simulink model "sim_battery_testrack_"  (R2023a)
settings: configuration reference "SharedConfig" (kept outside this file)
undefined symbols (not defined in the file or in its folder): battery_builder_rtmsupport, gcbh
libraries: nesl_utility x14, GD_Batterymodel_6_lib x8, fl_lib x7, BatteryCurrentManagement x1, batt_lib x1, BatteryBalancing x1, simulink x1, SimscapeFluids_lib x1
(part 1 of 2)
settings Model: Creator=DM  LastModifiedBy=ga84jar
settings ConfigSetRef: SourceName=SharedConfig  SourceLocation=Base Workspace

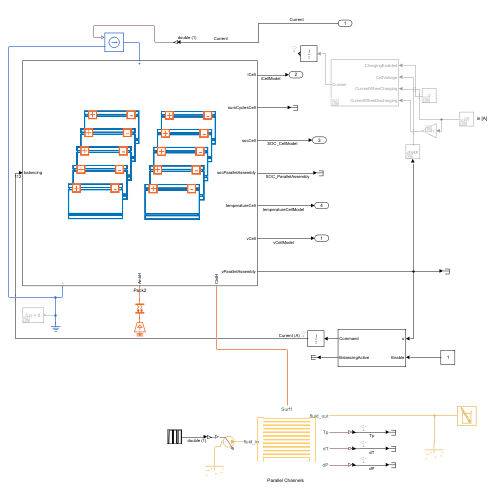
[thumbnail: Simulink's stored preview of the top-level diagram]
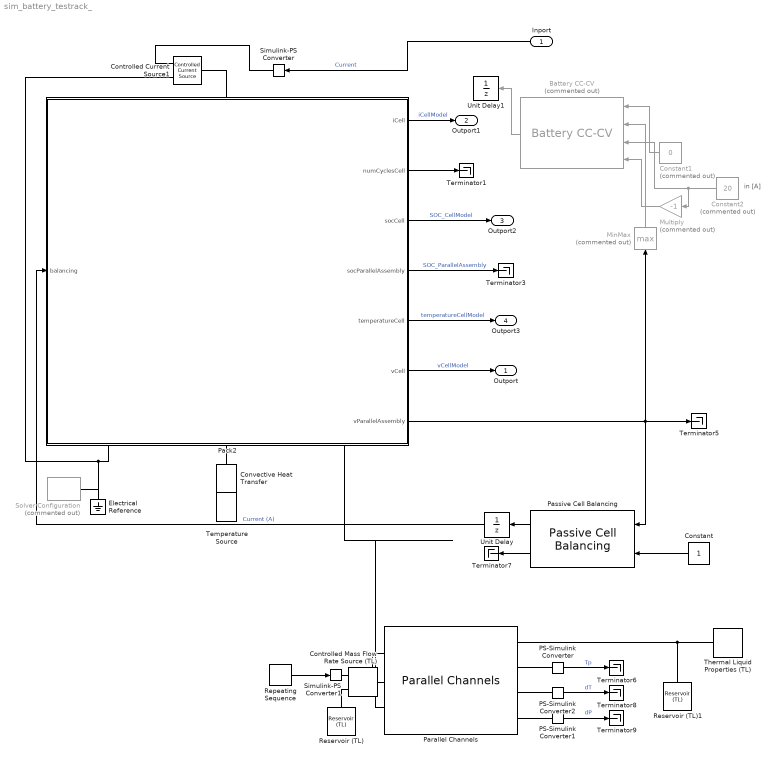
== system sim_battery_testrack_ ==
  note: in [A]
  Inport : Inport
  Battery CC-CV : BatteryCurrentManagement/Battery CC-CV  Commented=on  MaxCellVoltage=4.5  Kp=100  Ki=10  Kaw=1  Kt=1  Ts=-1
      settings: LibrarySourceBlock=batt_sl_lib/Current Management/Battery CC-CV
  Constant : Constant
  Constant1 : Constant  Commented=on  Value=0
  Constant2 : Constant  Commented=on  Value=20
  Controlled Current Source1 : fl_lib/Electrical/Electrical Sources/Controlled Current Source
  Controlled Mass Flow Rate Source (TL) : fl_lib/Thermal Liquid/Sources/Controlled Mass Flow Rate Source (TL)  power_spec=foundation.enum.power_spec.isentropic  area=0.01 m^2
      settings: InternalSimscapePortConfiguration="{\"Bottom\":[],\"Left\":[{\"id\":\"A\",\"label\":\"A\",\"type\":\"foundation.thermal_liquid.thermal_liquid\"},{\"id\":\"M\",\"label\":\"M\",\"type\":\"input\"}],\"Right\":[{\"id\":\"B\",\"label\":\"B\",\"type\":\"foundation.thermal_liquid.thermal_liquid\"}],\"Top\":[]}"
  Convective Heat Transfer : fl_lib/Thermal/Thermal Elements/Convective Heat Transfer  thermal_type=foundation.enum.constant_variable.constant  area=1e-4 m^2  heat_tr_coeff=20 W/(K*m^2)  min_heat_tr_coeff=1e-3 W/(K*m^2)  T_specify=off  T_priority=None  T=0 K  T_nominal_specify=off  T_nominal_unit=K  T_nominal_value=1  Q_specify=off  Q_priority=None  Q=0 W  Q_nominal_specify=off  Q_nominal_unit=W  Q_nominal_value=1
  Electrical Reference : fl_lib/Electrical/Electrical Elements/Electrical Reference
  MinMax : MinMax  Commented=on  Function=max
  Multiply : Gain  Commented=on  Gain=-1
  PS-Simulink Converter : nesl_utility/PS-Simulink Converter  PhysicalDomain=network_engine_domain  SubClassName=ps_output  LeftPortType=input  RightPortType=output  PseudoPeriodic=off  Frequencies=[]  VectorFormat=inherit  Unit=inherit  AffineConversion=off
  PS-Simulink Converter1 : nesl_utility/PS-Simulink Converter  PhysicalDomain=network_engine_domain  SubClassName=ps_output  LeftPortType=input  RightPortType=output  PseudoPeriodic=off  Frequencies=[]  VectorFormat=inherit  Unit=inherit  AffineConversion=off
  PS-Simulink Converter2 : nesl_utility/PS-Simulink Converter  PhysicalDomain=network_engine_domain  SubClassName=ps_output  LeftPortType=input  RightPortType=output  PseudoPeriodic=off  Frequencies=[]  VectorFormat=inherit  Unit=inherit  AffineConversion=off
  Pack2 : Subsystem  LoadFcn=battery_builder_rtmsupport('loadfcn',gcbh);
      settings: CopyFcn=battery_builder_rtmsupport('copyfcn',gcbh);  PreCopyFcn=battery_builder_rtmsupport('precopyfcn',gcbh);  PreDeleteFcn=battery_builder_rtmsupport('predeletefcn',gcbh);  PortSchema="{\"entries\":[{\"content\":{\"sides\":[{\"content\":{\"connectorIds\":[\"LConn1\"]},\"type\":\"ConnectorPlacement.EquallySpacedRectSide\",\"uuid\":\"eaf430c6-d28e-4a62-8b49-4d37c8edca5f\"},{\"content\":{\"connectorIds\":[\"RConn1\",\"RConn2\",\"RConn3\"],\"side\":\"RIGHT\"},\"type\":\"ConnectorPlacement.EquallySpacedRectSide\",\"uuid\":\"a95fddc1-7334-484a-9b4b-2e1f2360c9bb\"},{\"content\":{\"connectorIds\":[\"In1\"],\"side\":\"TOP\"},\"type\":\"ConnectorPlacement.EquallySpacedRectSide\",\"uuid\":\"f8c05a41-d443-4265-a433-e5e7047f73b2\"},{\"content\":{\"connectorIds\":[\"Out1\",\"Out2\",\"Out3\",\"Out4\",\"Out5\",\"Out6\",\"Out7\"],\"side\":\"BOTTOM\"},\"type\":\"ConnectorPlacement.EquallySpacedRectSide\",\"uuid\":\"9eaec147-65ce-4588-accb-be47b4d057de\"}]},\"type\":\"ConnectorPlacement.EquallySpacedConnector\",\"uuid\":\"9deafdf2-66e7-49dd-9ff8-5fa03867202c\"}],\"packageUris\":[\"http://schema.mathworks.com/mf0/Connector/R2020b\"],\"version\":\"1.0\"}"
      mask Display: image('$imagefile')
  Parallel Channels : batt_lib/Thermal/Parallel Channels  plateConnectivity=simscape.battery.enum.thermal.coolingPlateConnectivity.singleSided  numBattThermalNodes1=1  dimensionThermalNodes1=ones(1, 2)  locationThermalNodes1=ones(1, 2)  numBattThermalNodes2=1  dimensionThermalNodes2=ones(1, 2)  locationThermalNodes2=ones(1, 2)  plateDimX=2  plateDimY=5  plateTh=2e-3 m  plateThCond=20 W/(K*m)  plateDen=2500 kg/m^3  plateCp=447 J/(K*kg)  plateTemp_ini=300 K  Re_lam=2000  Re_tur=4000  Nu_lam=3.66  length_add=1e-3 m  shape_factor=64  nChannels=4  selectChannelOrientation=simscape.battery.enum.thermal.coolingChannelsDirection.alongX  channelDia=0.005 m  distributorDia=0.005 m  roughnessPipe=1.5e-05 m
      settings: InternalSimscapePortConfiguration="{\"Bottom\":[],\"Left\":[{\"id\":\"fluid_in\",\"label\":\"fluid_in\",\"type\":\"foundation.thermal_liquid.thermal_liquid\"}],\"Right\":[{\"id\":\"fluid_out\",\"label\":\"fluid_out\",\"type\":\"foundation.thermal_liquid.thermal_liquid\"},{\"id\":\"plotPlateT\",\"label\":\"Tp\",\"type\":\"output\"},{\"id\":\"tempSensor\",\"label\":\"dT\",\"type\":\"output\"},{\"id\":\"presSensor\",\"label\":\"dP\",\"type\":\"output\"}],\"Top\":[{\"id\":\"Side1\",\"label\":\"Surf1\",\"type\":\"foundation.thermal.thermal\"}]}"
  Passive Cell Balancing : BatteryBalancing/Passive Cell Balancing  Threshold=0.2  Td_on=1  Td_off=1  Ts=-1  dataType=double
      settings: LibrarySourceBlock=batt_sl_lib/Cell Balancing/Passive Cell Balancing
  Repeating Sequence : simulink/Sources/Repeating Sequence  rep_seq_t=[0 500 550 2001]  rep_seq_y=[0.00 0.00 0.01 0.01]
  Reservoir (TL) : fl_lib/Thermal Liquid/Elements/Reservoir (TL)  pressure_spec=foundation.enum.pressure_spec.atmospheric  reservoir_pressure=0.101325 MPa  reservoir_temperature=293.15 K  area=0.01 m^2
  Reservoir (TL)1 : fl_lib/Thermal Liquid/Elements/Reservoir (TL)  pressure_spec=foundation.enum.pressure_spec.atmospheric  reservoir_pressure=0.101325 MPa  reservoir_temperature=293.15 K  area=0.01 m^2
  Simulink-PS Converter : nesl_utility/Simulink-PS Converter  PhysicalDomain=network_engine_domain  SubClassName=ps_input  LeftPortType=input  RightPortType=output  PseudoPeriodic=off  Frequencies=[]  NoiseDistribution=none  NoiseParameters=[]  Unit=1  AffineConversion=off  FilteringAndDerivatives=provide  SimscapeFilterOrder=1  InputFilterTimeConstant=0.001  UdotUserProvided=0
  Simulink-PS Converter1 : nesl_utility/Simulink-PS Converter  PhysicalDomain=network_engine_domain  SubClassName=ps_input  LeftPortType=input  RightPortType=output  PseudoPeriodic=off  Frequencies=[]  NoiseDistribution=none  NoiseParameters=[]  Unit=1  AffineConversion=off  FilteringAndDerivatives=provide  SimscapeFilterOrder=1  InputFilterTimeConstant=0.001  UdotUserProvided=0
  Solver Configuration : nesl_utility/Solver Configuration  Commented=on  PhysicalDomain=network_engine_domain  SubClassName=solver  LeftPortType=input  RightPortType=generic  Tones=[]  Harmonics=[]  SimulateNoise=off  Profile=off  UseLocalSampling=off  EnableSwitchedLinearOptims=on  FrequencyDomain=off  UseCCode=off  RelTol=0.001  AbsTol=0.001  MinStep=1e-09  ToWorkspace=off  RevertToSquareIcSolve=off  NumHomotopyIterations=100  PhasorMode=off  PhasorModeNumHarmonics=1  ConsistencySolver=NEWTON_XTOL_AFTER_FTOL  IndexReductionMethod=DerivativeReplacement  DoDC=off  ResidualTolerance=1e-09  ConsistencyTolSource=GLOBAL  ConsistencyAbsTol=0.001  ConsistencyRelTol=0.001  ConsistencyTolFactor=0.001  UseLocalSolver=on  LocalSolverChoice=NE_BACKWARD_EULER_ADVANCER  ResolveIndetEquations=on  FunctionEvalNumThread=1  LocalSolverSampleTime=1  DoFixedCost=on  MaxNonlinIter=3  MaxModeIter=2  ComputeImpulses=off  ImpulseIterations=2  LinearAlgebra=auto  LinearAlgebraNumThread=0  EquationFormulation=NE_TIME_EF  DelaysMemoryBudget=51200  AutomaticFiltering=on  FilteringTimeConstant=0.001  PartitionStorageMethod=AS_NEEDED  PartitionMemoryBudget=1024  PartitionMethod=ROBUST
  Temperature Source : fl_lib/Thermal/Thermal Sources/Temperature Source  temperature=273.15+25 K
  Terminator{1,3,5..9} (7 alike) : Terminator
  Thermal Liquid Properties (TL) : SimscapeFluids_lib/Thermal Liquid/Utilities/Thermal Liquid Properties (TL)  fluid_list=fluids.thermal_liquid.utilities.enum.thermal_liquid_fluid_list.water  concentration_param_EG=fluids.thermal_liquid.utilities.enum.thermal_liquid_concentration.volume_fraction  concentration_param_PG=fluids.thermal_liquid.utilities.enum.thermal_liquid_concentration.volume_fraction  c_mass_SW=3.5e-3  c_mass_EG=0.1  c_mass_PG=0.1  c_mass_GL=0.1  c_vol_EG=0.1  c_vol_PG=0.1  beta_const_EG=2.1791 GPa  beta_const_PG=2.1791 GPa  beta_const_GL=2.1791 GPa  p_min_EG=0.01 MPa  p_min_PG=0.01 MPa  p_min_GL=0.01 MPa  p_max_EG=50 MPa  p_max_PG=50 MPa  p_max_GL=50 MPa  p_atm=0.101325 MPa  properties_range_check=simscape.enum.assert.action.error
  Unit Delay : UnitDelay  SampleTime=-1  HasFrameUpgradeWarning=on
  Unit Delay1 : UnitDelay  SampleTime=-1  HasFrameUpgradeWarning=on
  Outport : Outport
  Outport1 : Outport  Port=2
  Outport2 : Outport  Port=3
  Outport3 : Outport  Port=4
  wires:
  Pack2/1(iCell) -> Outport1/1  "iCellModel"
  Pack2/2(numCyclesCell) -> Terminator1/1
  Pack2/3(socCell) -> Outport2/1  "SOC_CellModel"
  Pack2/4(socParallelAssembly) -> Terminator3/1  "SOC_ParallelAssembly"
  Pack2/5(temperatureCell) -> Outport3/1  "temperatureCellModel"
  Pack2/6(vCell) -> Outport/1  "vCellModel"
  Passive Cell Balancing/2 -> Terminator7/1
  Constant/1 -> Passive Cell Balancing/2
  Constant1/1 -> Battery CC-CV/1
  Constant2/1 -> Multiply/1, Battery CC-CV/3
  Multiply/1 -> Battery CC-CV/4
  MinMax/1 -> Battery CC-CV/2
  Passive Cell Balancing/1 -> Unit Delay/1
  Unit Delay/1 -> Pack2/1(balancing)  "Current (A)"
  PS-Simulink Converter/1 -> Terminator6/1  "Tp"
  PS-Simulink Converter2/1 -> Terminator8/1  "dT"
  PS-Simulink Converter1/1 -> Terminator9/1  "dP"
  Repeating Sequence/1 -> Simulink-PS Converter1/1
  Inport/1 -> Simulink-PS Converter/1  "Current"
  Pack2/7(vParallelAssembly) -> Terminator5/1, Passive Cell Balancing/1, MinMax/1
  Battery CC-CV/1 -> Unit Delay1/1
  connections:
  Pack2/LConn1 -- Controlled Current Source1/LConn1
  Controlled Current Source1/RConn2 -- Pack2/RConn1 -- Electrical Reference/LConn1 -- Solver Configuration/RConn1
  Simulink-PS Converter/RConn1 -- Controlled Current Source1/RConn1
  Pack2/RConn3 -- Parallel Channels/LConn2
  PS-Simulink Converter/LConn1 -- Parallel Channels/RConn2
  PS-Simulink Converter2/LConn1 -- Parallel Channels/RConn3
  Parallel Channels/RConn4 -- PS-Simulink Converter1/LConn1
  Controlled Mass Flow Rate Source (TL)/RConn1 -- Parallel Channels/LConn1
  Simulink-PS Converter1/RConn1 -- Controlled Mass Flow Rate Source (TL)/LConn2
  Reservoir (TL)/LConn1 -- Controlled Mass Flow Rate Source (TL)/LConn1
  Thermal Liquid Properties (TL)/RConn1 -- Parallel Channels/RConn1 -- Reservoir (TL)1/LConn1
  Pack2/RConn2 -- Convective Heat Transfer/LConn1
  Temperature Source/LConn1 -- Convective Heat Transfer/RConn1

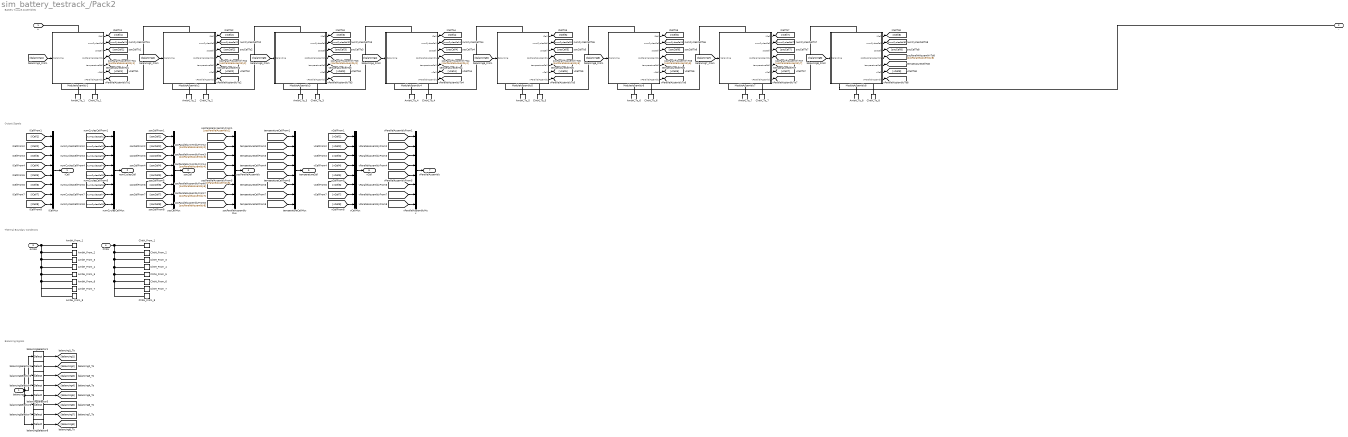
== system sim_battery_testrack_/Pack2 ==
  note: Battery Module Assemblies
  note: Output Signals
  note: Thermal Boundary Conditions
  note: Balancing Signals
  balancing : Inport  PortDimensions=112
  AmbH_From_1 : ConnectionLabel  Label=ambH_1
  AmbH_From_2 : ConnectionLabel  Label=ambH_2
  AmbH_From_3 : ConnectionLabel  Label=ambH_3
  AmbH_From_4 : ConnectionLabel  Label=ambH_4
  AmbH_From_5 : ConnectionLabel  Label=ambH_5
  AmbH_From_6 : ConnectionLabel  Label=ambH_6
  AmbH_From_7 : ConnectionLabel  Label=ambH_7
  AmbH_From_8 : ConnectionLabel  Label=ambH_8
  AmbH_To_1 : ConnectionLabel  Label=ambH_1
  AmbH_To_2 : ConnectionLabel  Label=ambH_2
  AmbH_To_3 : ConnectionLabel  Label=ambH_3
  AmbH_To_4 : ConnectionLabel  Label=ambH_4
  AmbH_To_5 : ConnectionLabel  Label=ambH_5
  AmbH_To_6 : ConnectionLabel  Label=ambH_6
  AmbH_To_7 : ConnectionLabel  Label=ambH_7
  AmbH_To_8 : ConnectionLabel  Label=ambH_8
  ClntH_From_1 : ConnectionLabel  Label=clntH_1
  ClntH_From_2 : ConnectionLabel  Label=clntH_2
  ClntH_From_3 : ConnectionLabel  Label=clntH_3
  ClntH_From_4 : ConnectionLabel  Label=clntH_4
  ClntH_From_5 : ConnectionLabel  Label=clntH_5
  ClntH_From_6 : ConnectionLabel  Label=clntH_6
  ClntH_From_7 : ConnectionLabel  Label=clntH_7
  ClntH_From_8 : ConnectionLabel  Label=clntH_8
  ClntH_To_1 : ConnectionLabel  Label=clntH_1
  ClntH_To_2 : ConnectionLabel  Label=clntH_2
  ClntH_To_3 : ConnectionLabel  Label=clntH_3
  ClntH_To_4 : ConnectionLabel  Label=clntH_4
  ClntH_To_5 : ConnectionLabel  Label=clntH_5
  ClntH_To_6 : ConnectionLabel  Label=clntH_6
  ClntH_To_7 : ConnectionLabel  Label=clntH_7
  ClntH_To_8 : ConnectionLabel  Label=clntH_8
  ModuleAssembly1 : Subsystem  LoadFcn=battery_builder_rtmsupport('loadfcn',gcbh);
      settings: CopyFcn=battery_builder_rtmsupport('copyfcn',gcbh);  PreCopyFcn=battery_builder_rtmsupport('precopyfcn',gcbh);  PreDeleteFcn=battery_builder_rtmsupport('predeletefcn',gcbh);  PortSchema="{\"entries\":[{\"content\":{\"sides\":[{\"content\":{\"connectorIds\":[\"LConn1\"]},\"type\":\"ConnectorPlacement.EquallySpacedRectSide\",\"uuid\":\"eaf430c6-d28e-4a62-8b49-4d37c8edca5f\"},{\"content\":{\"connectorIds\":[\"RConn1\",\"RConn2\",\"RConn3\"],\"side\":\"RIGHT\"},\"type\":\"ConnectorPlacement.EquallySpacedRectSide\",\"uuid\":\"a95fddc1-7334-484a-9b4b-2e1f2360c9bb\"},{\"content\":{\"connectorIds\":[\"In1\"],\"side\":\"TOP\"},\"type\":\"ConnectorPlacement.EquallySpacedRectSide\",\"uuid\":\"f8c05a41-d443-4265-a433-e5e7047f73b2\"},{\"content\":{\"connectorIds\":[\"Out1\",\"Out2\",\"Out3\",\"Out4\",\"Out5\",\"Out6\",\"Out7\"],\"side\":\"BOTTOM\"},\"type\":\"ConnectorPlacement.EquallySpacedRectSide\",\"uuid\":\"17eedd60-d70f-4d8c-966d-c796b4172b11\"}]},\"type\":\"ConnectorPlacement.EquallySpacedConnector\",\"uuid\":\"9deafdf2-66e7-49dd-9ff8-5fa03867202c\"}],\"packageUris\":[\"http://schema.mathworks.com/mf0/Connector/R2020b\"],\"version\":\"1.0\"}"
      mask Display: image('$imagefile')
  ModuleAssembly2 : Subsystem  LoadFcn=battery_builder_rtmsupport('loadfcn',gcbh);
      settings: CopyFcn=battery_builder_rtmsupport('copyfcn',gcbh);  PreCopyFcn=battery_builder_rtmsupport('precopyfcn',gcbh);  PreDeleteFcn=battery_builder_rtmsupport('predeletefcn',gcbh);  PortSchema="{\"entries\":[{\"content\":{\"sides\":[{\"content\":{\"connectorIds\":[\"LConn1\"]},\"type\":\"ConnectorPlacement.EquallySpacedRectSide\",\"uuid\":\"eaf430c6-d28e-4a62-8b49-4d37c8edca5f\"},{\"content\":{\"connectorIds\":[\"RConn1\",\"RConn2\",\"RConn3\"],\"side\":\"RIGHT\"},\"type\":\"ConnectorPlacement.EquallySpacedRectSide\",\"uuid\":\"a95fddc1-7334-484a-9b4b-2e1f2360c9bb\"},{\"content\":{\"connectorIds\":[\"In1\"],\"side\":\"TOP\"},\"type\":\"ConnectorPlacement.EquallySpacedRectSide\",\"uuid\":\"f8c05a41-d443-4265-a433-e5e7047f73b2\"},{\"content\":{\"connectorIds\":[\"Out1\",\"Out2\",\"Out3\",\"Out4\",\"Out5\",\"Out6\",\"Out7\"],\"side\":\"BOTTOM\"},\"type\":\"ConnectorPlacement.EquallySpacedRectSide\",\"uuid\":\"17eedd60-d70f-4d8c-966d-c796b4172b11\"}]},\"type\":\"ConnectorPlacement.EquallySpacedConnector\",\"uuid\":\"9deafdf2-66e7-49dd-9ff8-5fa03867202c\"}],\"packageUris\":[\"http://schema.mathworks.com/mf0/Connector/R2020b\"],\"version\":\"1.0\"}"
      mask Display: image('$imagefile')
  ModuleAssembly3 : Subsystem  LoadFcn=battery_builder_rtmsupport('loadfcn',gcbh);
      settings: CopyFcn=battery_builder_rtmsupport('copyfcn',gcbh);  PreCopyFcn=battery_builder_rtmsupport('precopyfcn',gcbh);  PreDeleteFcn=battery_builder_rtmsupport('predeletefcn',gcbh);  PortSchema="{\"entries\":[{\"content\":{\"sides\":[{\"content\":{\"connectorIds\":[\"LConn1\"]},\"type\":\"ConnectorPlacement.EquallySpacedRectSide\",\"uuid\":\"eaf430c6-d28e-4a62-8b49-4d37c8edca5f\"},{\"content\":{\"connectorIds\":[\"RConn1\",\"RConn2\",\"RConn3\"],\"side\":\"RIGHT\"},\"type\":\"ConnectorPlacement.EquallySpacedRectSide\",\"uuid\":\"a95fddc1-7334-484a-9b4b-2e1f2360c9bb\"},{\"content\":{\"connectorIds\":[\"In1\"],\"side\":\"TOP\"},\"type\":\"ConnectorPlacement.EquallySpacedRectSide\",\"uuid\":\"f8c05a41-d443-4265-a433-e5e7047f73b2\"},{\"content\":{\"connectorIds\":[\"Out1\",\"Out2\",\"Out3\",\"Out4\",\"Out5\",\"Out6\",\"Out7\"],\"side\":\"BOTTOM\"},\"type\":\"ConnectorPlacement.EquallySpacedRectSide\",\"uuid\":\"17eedd60-d70f-4d8c-966d-c796b4172b11\"}]},\"type\":\"ConnectorPlacement.EquallySpacedConnector\",\"uuid\":\"9deafdf2-66e7-49dd-9ff8-5fa03867202c\"}],\"packageUris\":[\"http://schema.mathworks.com/mf0/Connector/R2020b\"],\"version\":\"1.0\"}"
      mask Display: image('$imagefile')
  ModuleAssembly4 : Subsystem  LoadFcn=battery_builder_rtmsupport('loadfcn',gcbh);
      settings: CopyFcn=battery_builder_rtmsupport('copyfcn',gcbh);  PreCopyFcn=battery_builder_rtmsupport('precopyfcn',gcbh);  PreDeleteFcn=battery_builder_rtmsupport('predeletefcn',gcbh);  PortSchema="{\"entries\":[{\"content\":{\"sides\":[{\"content\":{\"connectorIds\":[\"LConn1\"]},\"type\":\"ConnectorPlacement.EquallySpacedRectSide\",\"uuid\":\"eaf430c6-d28e-4a62-8b49-4d37c8edca5f\"},{\"content\":{\"connectorIds\":[\"RConn1\",\"RConn2\",\"RConn3\"],\"side\":\"RIGHT\"},\"type\":\"ConnectorPlacement.EquallySpacedRectSide\",\"uuid\":\"a95fddc1-7334-484a-9b4b-2e1f2360c9bb\"},{\"content\":{\"connectorIds\":[\"In1\"],\"side\":\"TOP\"},\"type\":\"ConnectorPlacement.EquallySpacedRectSide\",\"uuid\":\"f8c05a41-d443-4265-a433-e5e7047f73b2\"},{\"content\":{\"connectorIds\":[\"Out1\",\"Out2\",\"Out3\",\"Out4\",\"Out5\",\"Out6\",\"Out7\"],\"side\":\"BOTTOM\"},\"type\":\"ConnectorPlacement.EquallySpacedRectSide\",\"uuid\":\"17eedd60-d70f-4d8c-966d-c796b4172b11\"}]},\"type\":\"ConnectorPlacement.EquallySpacedConnector\",\"uuid\":\"9deafdf2-66e7-49dd-9ff8-5fa03867202c\"}],\"packageUris\":[\"http://schema.mathworks.com/mf0/Connector/R2020b\"],\"version\":\"1.0\"}"
      mask Display: image('$imagefile')
  ModuleAssembly5 : Subsystem  LoadFcn=battery_builder_rtmsupport('loadfcn',gcbh);
      settings: CopyFcn=battery_builder_rtmsupport('copyfcn',gcbh);  PreCopyFcn=battery_builder_rtmsupport('precopyfcn',gcbh);  PreDeleteFcn=battery_builder_rtmsupport('predeletefcn',gcbh);  PortSchema="{\"entries\":[{\"content\":{\"sides\":[{\"content\":{\"connectorIds\":[\"LConn1\"]},\"type\":\"ConnectorPlacement.EquallySpacedRectSide\",\"uuid\":\"eaf430c6-d28e-4a62-8b49-4d37c8edca5f\"},{\"content\":{\"connectorIds\":[\"RConn1\",\"RConn2\",\"RConn3\"],\"side\":\"RIGHT\"},\"type\":\"ConnectorPlacement.EquallySpacedRectSide\",\"uuid\":\"a95fddc1-7334-484a-9b4b-2e1f2360c9bb\"},{\"content\":{\"connectorIds\":[\"In1\"],\"side\":\"TOP\"},\"type\":\"ConnectorPlacement.EquallySpacedRectSide\",\"uuid\":\"f8c05a41-d443-4265-a433-e5e7047f73b2\"},{\"content\":{\"connectorIds\":[\"Out1\",\"Out2\",\"Out3\",\"Out4\",\"Out5\",\"Out6\",\"Out7\"],\"side\":\"BOTTOM\"},\"type\":\"ConnectorPlacement.EquallySpacedRectSide\",\"uuid\":\"17eedd60-d70f-4d8c-966d-c796b4172b11\"}]},\"type\":\"ConnectorPlacement.EquallySpacedConnector\",\"uuid\":\"9deafdf2-66e7-49dd-9ff8-5fa03867202c\"}],\"packageUris\":[\"http://schema.mathworks.com/mf0/Connector/R2020b\"],\"version\":\"1.0\"}"
      mask Display: image('$imagefile')
  ModuleAssembly6 : Subsystem  LoadFcn=battery_builder_rtmsupport('loadfcn',gcbh);
      settings: CopyFcn=battery_builder_rtmsupport('copyfcn',gcbh);  PreCopyFcn=battery_builder_rtmsupport('precopyfcn',gcbh);  PreDeleteFcn=battery_builder_rtmsupport('predeletefcn',gcbh);  PortSchema="{\"entries\":[{\"content\":{\"sides\":[{\"content\":{\"connectorIds\":[\"LConn1\"]},\"type\":\"ConnectorPlacement.EquallySpacedRectSide\",\"uuid\":\"eaf430c6-d28e-4a62-8b49-4d37c8edca5f\"},{\"content\":{\"connectorIds\":[\"RConn1\",\"RConn2\",\"RConn3\"],\"side\":\"RIGHT\"},\"type\":\"ConnectorPlacement.EquallySpacedRectSide\",\"uuid\":\"a95fddc1-7334-484a-9b4b-2e1f2360c9bb\"},{\"content\":{\"connectorIds\":[\"In1\"],\"side\":\"TOP\"},\"type\":\"ConnectorPlacement.EquallySpacedRectSide\",\"uuid\":\"f8c05a41-d443-4265-a433-e5e7047f73b2\"},{\"content\":{\"connectorIds\":[\"Out1\",\"Out2\",\"Out3\",\"Out4\",\"Out5\",\"Out6\",\"Out7\"],\"side\":\"BOTTOM\"},\"type\":\"ConnectorPlacement.EquallySpacedRectSide\",\"uuid\":\"17eedd60-d70f-4d8c-966d-c796b4172b11\"}]},\"type\":\"ConnectorPlacement.EquallySpacedConnector\",\"uuid\":\"9deafdf2-66e7-49dd-9ff8-5fa03867202c\"}],\"packageUris\":[\"http://schema.mathworks.com/mf0/Connector/R2020b\"],\"version\":\"1.0\"}"
      mask Display: image('$imagefile')
  ModuleAssembly7 : Subsystem  LoadFcn=battery_builder_rtmsupport('loadfcn',gcbh);
      settings: CopyFcn=battery_builder_rtmsupport('copyfcn',gcbh);  PreCopyFcn=battery_builder_rtmsupport('precopyfcn',gcbh);  PreDeleteFcn=battery_builder_rtmsupport('predeletefcn',gcbh);  PortSchema="{\"entries\":[{\"content\":{\"sides\":[{\"content\":{\"connectorIds\":[\"LConn1\"]},\"type\":\"ConnectorPlacement.EquallySpacedRectSide\",\"uuid\":\"eaf430c6-d28e-4a62-8b49-4d37c8edca5f\"},{\"content\":{\"connectorIds\":[\"RConn1\",\"RConn2\",\"RConn3\"],\"side\":\"RIGHT\"},\"type\":\"ConnectorPlacement.EquallySpacedRectSide\",\"uuid\":\"a95fddc1-7334-484a-9b4b-2e1f2360c9bb\"},{\"content\":{\"connectorIds\":[\"In1\"],\"side\":\"TOP\"},\"type\":\"ConnectorPlacement.EquallySpacedRectSide\",\"uuid\":\"f8c05a41-d443-4265-a433-e5e7047f73b2\"},{\"content\":{\"connectorIds\":[\"Out1\",\"Out2\",\"Out3\",\"Out4\",\"Out5\",\"Out6\",\"Out7\"],\"side\":\"BOTTOM\"},\"type\":\"ConnectorPlacement.EquallySpacedRectSide\",\"uuid\":\"17eedd60-d70f-4d8c-966d-c796b4172b11\"}]},\"type\":\"ConnectorPlacement.EquallySpacedConnector\",\"uuid\":\"9deafdf2-66e7-49dd-9ff8-5fa03867202c\"}],\"packageUris\":[\"http://schema.mathworks.com/mf0/Connector/R2020b\"],\"version\":\"1.0\"}"
      mask Display: image('$imagefile')
  ModuleAssembly8 : Subsystem  LoadFcn=battery_builder_rtmsupport('loadfcn',gcbh);
      settings: CopyFcn=battery_builder_rtmsupport('copyfcn',gcbh);  PreCopyFcn=battery_builder_rtmsupport('precopyfcn',gcbh);  PreDeleteFcn=battery_builder_rtmsupport('predeletefcn',gcbh);  PortSchema="{\"entries\":[{\"content\":{\"sides\":[{\"content\":{\"connectorIds\":[\"LConn1\"]},\"type\":\"ConnectorPlacement.EquallySpacedRectSide\",\"uuid\":\"eaf430c6-d28e-4a62-8b49-4d37c8edca5f\"},{\"content\":{\"connectorIds\":[\"RConn1\",\"RConn2\",\"RConn3\"],\"side\":\"RIGHT\"},\"type\":\"ConnectorPlacement.EquallySpacedRectSide\",\"uuid\":\"a95fddc1-7334-484a-9b4b-2e1f2360c9bb\"},{\"content\":{\"connectorIds\":[\"In1\"],\"side\":\"TOP\"},\"type\":\"ConnectorPlacement.EquallySpacedRectSide\",\"uuid\":\"f8c05a41-d443-4265-a433-e5e7047f73b2\"},{\"content\":{\"connectorIds\":[\"Out1\",\"Out2\",\"Out3\",\"Out4\",\"Out5\",\"Out6\",\"Out7\"],\"side\":\"BOTTOM\"},\"type\":\"ConnectorPlacement.EquallySpacedRectSide\",\"uuid\":\"17eedd60-d70f-4d8c-966d-c796b4172b11\"}]},\"type\":\"ConnectorPlacement.EquallySpacedConnector\",\"uuid\":\"9deafdf2-66e7-49dd-9ff8-5fa03867202c\"}],\"packageUris\":[\"http://schema.mathworks.com/mf0/Connector/R2020b\"],\"version\":\"1.0\"}"
      mask Display: image('$imagefile')
  balancingSelector1 : Selector  InputPortWidth=112  IndexOptions=Index vector (dialog)  Indices="[1   2   3   4   5   6   7   8   9  10  11  12  13  14]"  OutputSizes=1
  balancingSelector2 : Selector  InputPortWidth=112  IndexOptions=Index vector (dialog)  Indices="[15  16  17  18  19  20  21  22  23  24  25  26  27  28]"  OutputSizes=1
  balancingSelector3 : Selector  InputPortWidth=112  IndexOptions=Index vector (dialog)  Indices="[29  30  31  32  33  34  35  36  37  38  39  40  41  42]"  OutputSizes=1
  balancingSelector4 : Selector  InputPortWidth=112  IndexOptions=Index vector (dialog)  Indices="[43  44  45  46  47  48  49  50  51  52  53  54  55  56]"  OutputSizes=1
  balancingSelector5 : Selector  InputPortWidth=112  IndexOptions=Index vector (dialog)  Indices="[57  58  59  60  61  62  63  64  65  66  67  68  69  70]"  OutputSizes=1
  balancingSelector6 : Selector  InputPortWidth=112  IndexOptions=Index vector (dialog)  Indices="[71  72  73  74  75  76  77  78  79  80  81  82  83  84]"  OutputSizes=1
  balancingSelector7 : Selector  InputPortWidth=112  IndexOptions=Index vector (dialog)  Indices="[85  86  87  88  89  90  91  92  93  94  95  96  97  98]"  OutputSizes=1
  balancingSelector8 : Selector  InputPortWidth=112  IndexOptions=Index vector (dialog)  Indices="[99  100  101  102  103  104  105  106  107  108  109  110  111  112]"  OutputSizes=1
  iCellMux : Mux  Inputs=8
  numCyclesCellMux : Mux  Inputs=8
  socCellMux : Mux  Inputs=8
  socParallelAssemblyMux : Mux  Inputs=8
  temperatureCellMux : Mux  Inputs=8
  vCellMux : Mux  Inputs=8
  vParallelAssemblyMux : Mux  Inputs=8
  + : PMIOPort  Side=Left
  - : PMIOPort  Port=2  Side=Right
  AmbH : PMIOPort  Port=3  Side=Right  ConnectionType=Connection: foundation.thermal.thermal
  ClntH : PMIOPort  Port=4  Side=Right  ConnectionType=Connection: foundation.thermal.thermal
  iCell : Outport
  numCyclesCell : Outport  Port=2
  socCell : Outport  Port=3
  socParallelAssembly : Outport  Port=4
  temperatureCell : Outport  Port=5
  vCell : Outport  Port=6
  vParallelAssembly : Outport  Port=7
  wires:
  ModuleAssembly1/1(iCell) -> [iCell1]
  iCellMux/1 -> iCell/1
  [iCell1] -> iCellMux/1
  ModuleAssembly1/2(numCyclesCell) -> [numCyclesCell1]
  numCyclesCellMux/1 -> numCyclesCell/1
  [numCyclesCell1] -> numCyclesCellMux/1
  ModuleAssembly1/3(socCell) -> [socCell1]
  socCellMux/1 -> socCell/1
  [socCell1] -> socCellMux/1
  ModuleAssembly1/4(socParallelAssembly) -> [socParallelAssembly1]
  socParallelAssemblyMux/1 -> socParallelAssembly/1
  [socParallelAssembly1] -> socParallelAssemblyMux/1
  ModuleAssembly1/5(temperatureCell) -> [temperatureCell1]
  temperatureCellMux/1 -> temperatureCell/1
  [temperatureCell1] -> temperatureCellMux/1
  ModuleAssembly1/6(vCell) -> [vCell1]
  vCellMux/1 -> vCell/1
  [vCell1] -> vCellMux/1
  ModuleAssembly1/7(vParallelAssembly) -> [vParallelAssembly1]
  vParallelAssemblyMux/1 -> vParallelAssembly/1
  [vParallelAssembly1] -> vParallelAssemblyMux/1
  ModuleAssembly2/1(iCell) -> [iCell2]
  [iCell2] -> iCellMux/2
  ModuleAssembly2/2(numCyclesCell) -> [numCyclesCell2]
  [numCyclesCell2] -> numCyclesCellMux/2
  ModuleAssembly2/3(socCell) -> [socCell2]
  [socCell2] -> socCellMux/2
  ModuleAssembly2/4(socParallelAssembly) -> [socParallelAssembly2]
  [socParallelAssembly2] -> socParallelAssemblyMux/2
  ModuleAssembly2/5(temperatureCell) -> [temperatureCell2]
  [temperatureCell2] -> temperatureCellMux/2
  ModuleAssembly2/6(vCell) -> [vCell2]
  [vCell2] -> vCellMux/2
  ModuleAssembly2/7(vParallelAssembly) -> [vParallelAssembly2]
  [vParallelAssembly2] -> vParallelAssemblyMux/2
  ModuleAssembly3/1(iCell) -> [iCell3]
  [iCell3] -> iCellMux/3
  ModuleAssembly3/2(numCyclesCell) -> [numCyclesCell3]
  [numCyclesCell3] -> numCyclesCellMux/3
  ModuleAssembly3/3(socCell) -> [socCell3]
  [socCell3] -> socCellMux/3
  ModuleAssembly3/4(socParallelAssembly) -> [socParallelAssembly3]
  [socParallelAssembly3] -> socParallelAssemblyMux/3
  ModuleAssembly3/5(temperatureCell) -> [temperatureCell3]
  [temperatureCell3] -> temperatureCellMux/3
  ModuleAssembly3/6(vCell) -> [vCell3]
  [vCell3] -> vCellMux/3
  ModuleAssembly3/7(vParallelAssembly) -> [vParallelAssembly3]
  [vParallelAssembly3] -> vParallelAssemblyMux/3
  ModuleAssembly4/1(iCell) -> [iCell4]
  [iCell4] -> iCellMux/4
  ModuleAssembly4/2(numCyclesCell) -> [numCyclesCell4]
  [numCyclesCell4] -> numCyclesCellMux/4
  ModuleAssembly4/3(socCell) -> [socCell4]
  [socCell4] -> socCellMux/4
  ModuleAssembly4/4(socParallelAssembly) -> [socParallelAssembly4]
  [socParallelAssembly4] -> socParallelAssemblyMux/4
  ModuleAssembly4/5(temperatureCell) -> [temperatureCell4]
  [temperatureCell4] -> temperatureCellMux/4
  ModuleAssembly4/6(vCell) -> [vCell4]
  [vCell4] -> vCellMux/4
  ModuleAssembly4/7(vParallelAssembly) -> [vParallelAssembly4]
  [vParallelAssembly4] -> vParallelAssemblyMux/4
  ModuleAssembly5/1(iCell) -> [iCell5]
  [iCell5] -> iCellMux/5
  ModuleAssembly5/2(numCyclesCell) -> [numCyclesCell5]
  [numCyclesCell5] -> numCyclesCellMux/5
  ModuleAssembly5/3(socCell) -> [socCell5]
  [socCell5] -> socCellMux/5
  ModuleAssembly5/4(socParallelAssembly) -> [socParallelAssembly5]
  [socParallelAssembly5] -> socParallelAssemblyMux/5
  ModuleAssembly5/5(temperatureCell) -> [temperatureCell5]
  [temperatureCell5] -> temperatureCellMux/5
  ModuleAssembly5/6(vCell) -> [vCell5]
  [vCell5] -> vCellMux/5
  ModuleAssembly5/7(vParallelAssembly) -> [vParallelAssembly5]
  [vParallelAssembly5] -> vParallelAssemblyMux/5
  ModuleAssembly6/1(iCell) -> [iCell6]
  [iCell6] -> iCellMux/6
  ModuleAssembly6/2(numCyclesCell) -> [numCyclesCell6]
  [numCyclesCell6] -> numCyclesCellMux/6
  ModuleAssembly6/3(socCell) -> [socCell6]
  [socCell6] -> socCellMux/6
  ModuleAssembly6/4(socParallelAssembly) -> [socParallelAssembly6]
  [socParallelAssembly6] -> socParallelAssemblyMux/6
  ModuleAssembly6/5(temperatureCell) -> [temperatureCell6]
  [temperatureCell6] -> temperatureCellMux/6
  ModuleAssembly6/6(vCell) -> [vCell6]
  [vCell6] -> vCellMux/6
  ModuleAssembly6/7(vParallelAssembly) -> [vParallelAssembly6]
  [vParallelAssembly6] -> vParallelAssemblyMux/6
  ModuleAssembly7/1(iCell) -> [iCell7]
  [iCell7] -> iCellMux/7
  ModuleAssembly7/2(numCyclesCell) -> [numCyclesCell7]
  [numCyclesCell7] -> numCyclesCellMux/7
  ModuleAssembly7/3(socCell) -> [socCell7]
  [socCell7] -> socCellMux/7
  ModuleAssembly7/4(socParallelAssembly) -> [socParallelAssembly7]
  [socParallelAssembly7] -> socParallelAssemblyMux/7
  ModuleAssembly7/5(temperatureCell) -> [temperatureCell7]
  [temperatureCell7] -> temperatureCellMux/7
  ModuleAssembly7/6(vCell) -> [vCell7]
  [vCell7] -> vCellMux/7
  ModuleAssembly7/7(vParallelAssembly) -> [vParallelAssembly7]
  [vParallelAssembly7] -> vParallelAssemblyMux/7
  ModuleAssembly8/1(iCell) -> [iCell8]
  [iCell8] -> iCellMux/8
  ModuleAssembly8/2(numCyclesCell) -> [numCyclesCell8]
  [numCyclesCell8] -> numCyclesCellMux/8
  ModuleAssembly8/3(socCell) -> [socCell8]
  [socCell8] -> socCellMux/8
  ModuleAssembly8/4(socParallelAssembly) -> [socParallelAssembly8]
  [socParallelAssembly8] -> socParallelAssemblyMux/8
  ModuleAssembly8/5(temperatureCell) -> [temperatureCell8]
  [temperatureCell8] -> temperatureCellMux/8
  ModuleAssembly8/6(vCell) -> [vCell8]
  [vCell8] -> vCellMux/8
  ModuleAssembly8/7(vParallelAssembly) -> [vParallelAssembly8]
  [vParallelAssembly8] -> vParallelAssemblyMux/8
  [balancing1] -> ModuleAssembly1/1(balancing)
  balancing/1 -> balancingSelector7/1, balancingSelector8/1, balancingSelector6/1, balancingSelector5/1, balancingSelector2/1, balancingSelector3/1, balancingSelector4/1, balancingSelector1/1
  balancingSelector1/1 -> [balancing1]
  [balancing2] -> ModuleAssembly2/1(balancing)
  balancingSelector2/1 -> [balancing2]
  [balancing3] -> ModuleAssembly3/1(balancing)
  balancingSelector3/1 -> [balancing3]
  [balancing4] -> ModuleAssembly4/1(balancing)
  balancingSelector4/1 -> [balancing4]
  [balancing5] -> ModuleAssembly5/1(balancing)
  balancingSelector5/1 -> [balancing5]
  [balancing6] -> ModuleAssembly6/1(balancing)
  balancingSelector6/1 -> [balancing6]
  [balancing7] -> ModuleAssembly7/1(balancing)
  balancingSelector7/1 -> [balancing7]
  [balancing8] -> ModuleAssembly8/1(balancing)
  balancingSelector8/1 -> [balancing8]
  connections:
  ModuleAssembly2/LConn1 -- ModuleAssembly1/RConn1
  ModuleAssembly3/LConn1 -- ModuleAssembly2/RConn1
  ModuleAssembly4/LConn1 -- ModuleAssembly3/RConn1
  ModuleAssembly5/LConn1 -- ModuleAssembly4/RConn1
  ModuleAssembly6/LConn1 -- ModuleAssembly5/RConn1
  ModuleAssembly7/LConn1 -- ModuleAssembly6/RConn1
  ModuleAssembly8/LConn1 -- ModuleAssembly7/RConn1
  ModuleAssembly1/LConn1 -- +/RConn1
  ModuleAssembly8/RConn1 -- -/RConn1
  AmbH_To_1/LConn1 -- ModuleAssembly1/RConn2
  AmbH_From_1/LConn1 -- AmbH_From_8/LConn1 -- AmbH_From_7/LConn1 -- AmbH_From_6/LConn1 -- AmbH_From_5/LConn1 -- AmbH_From_4/LConn1 -- AmbH_From_3/LConn1 -- AmbH_From_2/LConn1 -- AmbH/RConn1
  AmbH_To_2/LConn1 -- ModuleAssembly2/RConn2
  AmbH_To_3/LConn1 -- ModuleAssembly3/RConn2
  AmbH_To_4/LConn1 -- ModuleAssembly4/RConn2
  AmbH_To_5/LConn1 -- ModuleAssembly5/RConn2
  AmbH_To_6/LConn1 -- ModuleAssembly6/RConn2
  AmbH_To_7/LConn1 -- ModuleAssembly7/RConn2
  AmbH_To_8/LConn1 -- ModuleAssembly8/RConn2
  ClntH_To_1/LConn1 -- ModuleAssembly1/RConn3
  ClntH_From_1/LConn1 -- ClntH_From_8/LConn1 -- ClntH_From_7/LConn1 -- ClntH_From_6/LConn1 -- ClntH_From_5/LConn1 -- ClntH_From_4/LConn1 -- ClntH_From_3/LConn1 -- ClntH_From_2/LConn1 -- ClntH/RConn1
  ClntH_To_2/LConn1 -- ModuleAssembly2/RConn3
  ClntH_To_3/LConn1 -- ModuleAssembly3/RConn3
  ClntH_To_4/LConn1 -- ModuleAssembly4/RConn3
  ClntH_To_5/LConn1 -- ModuleAssembly5/RConn3
  ClntH_To_6/LConn1 -- ModuleAssembly6/RConn3
  ClntH_To_7/LConn1 -- ModuleAssembly7/RConn3
  ClntH_To_8/LConn1 -- ModuleAssembly8/RConn3

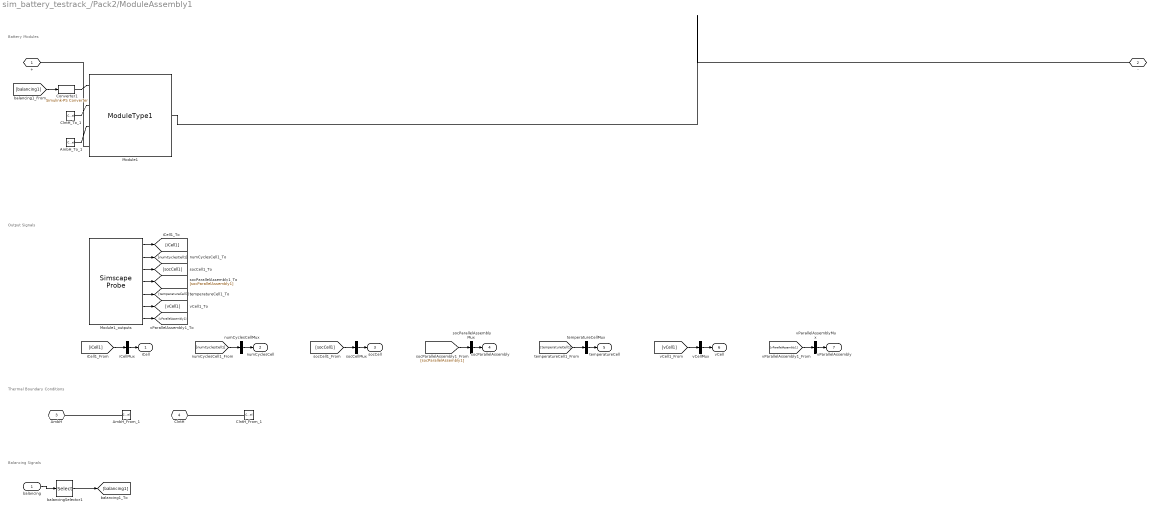
== system sim_battery_testrack_/Pack2/ModuleAssembly1 ==
  note: Balancing Signals
  note: Thermal Boundary Conditions
  note: Output Signals
  note: Battery Modules
  balancing : Inport  PortDimensions=14
  AmbH_From_1 : ConnectionLabel  Label=ambH_1
  AmbH_To_1 : ConnectionLabel  Label=ambH_1
  ClntH_From_1 : ConnectionLabel  Label=clntH_1
  ClntH_To_1 : ConnectionLabel  Label=clntH_1
  Converter1 : nesl_utility/Simulink-PS Converter  PhysicalDomain=network_engine_domain  SubClassName=ps_input  LeftPortType=input  RightPortType=output  PseudoPeriodic=off  Frequencies=[]  NoiseDistribution=none  NoiseParameters=[]  Unit=1  AffineConversion=off  FilteringAndDerivatives=provide  SimscapeFilterOrder=1  InputFilterTimeConstant=0.001  UdotUserProvided=0
  Module1 : GD_Batterymodel_6_lib/Modules/ModuleType1  SOC_vecCell=ModuleType1.SOC_vecCell  T_vecCell=ModuleType1.T_vecCell K  V0_matCell=ModuleType1.V0_matCell V  V_rangeCell=ModuleType1.V_rangeCell V  R0_matCell=ModuleType1.R0_matCell Ohm  AHCell=ModuleType1.AHCell A*hr  extrapolation_optionCell=simscape.enum.extrapolation.nearest  R1_matCell=ModuleType1.R1_matCell Ohm  tau1_matCell=ModuleType1.tau1_matCell s  R2_matCell=ModuleType1.R2_matCell Ohm  tau2_matCell=ModuleType1.tau2_matCell s  thermal_massCell=ModuleType1.thermal_massCell J/K  CoolantResistance=ModuleType1.CoolantResistance K/W  AmbientResistance=ModuleType1.AmbientResistance K/W  CellBalancingClosedResistance=ModuleType1.CellBalancingClosedResistance Ohm  CellBalancingOpenConductance=ModuleType1.CellBalancingOpenConductance 1/Ohm  CellBalancingThreshold=ModuleType1.CellBalancingThreshold  CellBalancingResistance=ModuleType1.CellBalancingResistance Ohm  P=3  S=14  iCell_specify=on  iCell_priority=None  iCell=ModuleAssembly1.Module1.iCell A  iCell_nominal_specify=off  iCell_nominal_unit=A  iCell_nominal_value=1  vCell_specify=on  vCell_priority=None  vCell=ModuleAssembly1.Module1.vCell V  vCell_nominal_specify=off  vCell_nominal_unit=V  vCell_nominal_value=1  socCell_specify=on  socCell_priority=High  socCell=ModuleAssembly1.Module1.socCell  socCell_nominal_specify=off  socCell_nominal_unit=1  socCell_nominal_value=1  numCyclesCell_specify=on  numCyclesCell_priority=High  numCyclesCell=ModuleAssembly1.Module1.numCyclesCell  numCyclesCell_nominal_specify=off  numCyclesCell_nominal_unit=1  numCyclesCell_nominal_value=1  temperatureCell_specify=on  temperatureCell_priority=High  temperatureCell=ModuleAssembly1.Module1.temperatureCell K  temperatureCell_nominal_specify=off  temperatureCell_nominal_unit=K  temperatureCell_nominal_value=1  vParallelAssembly_specify=on  vParallelAssembly_priority=None  vParallelAssembly=ModuleAssembly1.Module1.vParallelAssembly V  vParallelAssembly_nominal_specify=off  vParallelAssembly_nominal_unit=V  vParallelAssembly_nominal_value=1  socParallelAssembly_specify=on  socParallelAssembly_priority=None  socParallelAssembly=ModuleAssembly1.Module1.socParallelAssembly  socParallelAssembly_nominal_specify=off  socParallelAssembly_nominal_unit=1  socParallelAssembly_nominal_value=1
      settings: InternalSimscapePortConfiguration="{\"Bottom\":[{\"id\":\"n\",\"label\":\"-\",\"type\":\"foundation.electrical.electrical\"}],\"Left\":[{\"id\":\"enableCellBalancing\",\"label\":\"CB\",\"type\":\"input\"},{\"id\":\"ClntH\",\"label\":\"CH\",\"type\":\"foundation.thermal.thermal\"},{\"id\":\"AmbH\",\"label\":\"AH\",\"type\":\"foundation.thermal.thermal\"}],\"Right\":[],\"Top\":[{\"id\":\"p\",\"label\":\"+\",\"type\":\"foundation.electrical.electrical\"}]}"
  Module1_outputs : SimscapeProbe  BoundBlock=1380  Variables={iCell, numCyclesCell, socCell, socParallelAssembly, temperatureCell, vCell, vParallelAssembly}
  balancingSelector1 : Selector  InputPortWidth=14  IndexOptions=Index vector (dialog)  Indices="[1   2   3   4   5   6   7   8   9  10  11  12  13  14]"  OutputSizes=1
  iCellMux : Mux  Inputs=1
  numCyclesCellMux : Mux  Inputs=1
  socCellMux : Mux  Inputs=1
  socParallelAssemblyMux : Mux  Inputs=1
  temperatureCellMux : Mux  Inputs=1
  vCellMux : Mux  Inputs=1
  vParallelAssemblyMux : Mux  Inputs=1
  + : PMIOPort  Side=Left
  - : PMIOPort  Port=2  Side=Right
  AmbH : PMIOPort  Port=3  Side=Right  ConnectionType=Connection: foundation.thermal.thermal
  ClntH : PMIOPort  Port=4  Side=Right  ConnectionType=Connection: foundation.thermal.thermal
  iCell : Outport
  numCyclesCell : Outport  Port=2
  socCell : Outport  Port=3
  socParallelAssembly : Outport  Port=4
  temperatureCell : Outport  Port=5
  vCell : Outport  Port=6
  vParallelAssembly : Outport  Port=7
  wires:
  balancingSelector1/1 -> [balancing1]
  balancing/1 -> balancingSelector1/1
  [balancing1] -> Converter1/1
  [vParallelAssembly1] -> vParallelAssemblyMux/1
  vParallelAssemblyMux/1 -> vParallelAssembly/1
  Module1_outputs/7 -> [vParallelAssembly1]
  [vCell1] -> vCellMux/1
  vCellMux/1 -> vCell/1
  Module1_outputs/6 -> [vCell1]
  [temperatureCell1] -> temperatureCellMux/1
  temperatureCellMux/1 -> temperatureCell/1
  Module1_outputs/5 -> [temperatureCell1]
  [socParallelAssembly1] -> socParallelAssemblyMux/1
  socParallelAssemblyMux/1 -> socParallelAssembly/1
  Module1_outputs/4 -> [socParallelAssembly1]
  [socCell1] -> socCellMux/1
  socCellMux/1 -> socCell/1
  Module1_outputs/3 -> [socCell1]
  [numCyclesCell1] -> numCyclesCellMux/1
  numCyclesCellMux/1 -> numCyclesCell/1
  Module1_outputs/2 -> [numCyclesCell1]
  [iCell1] -> iCellMux/1
  iCellMux/1 -> iCell/1
  Module1_outputs/1 -> [iCell1]
  connections:
  Converter1/RConn1 -- Module1/LConn1
  ClntH_From_1/LConn1 -- ClntH/RConn1
  ClntH_To_1/LConn1 -- Module1/LConn2
  AmbH_From_1/LConn1 -- AmbH/RConn1
  AmbH_To_1/LConn1 -- Module1/LConn3
  Module1/RConn1 -- -/RConn1
  Module1/LConn4 -- +/RConn1

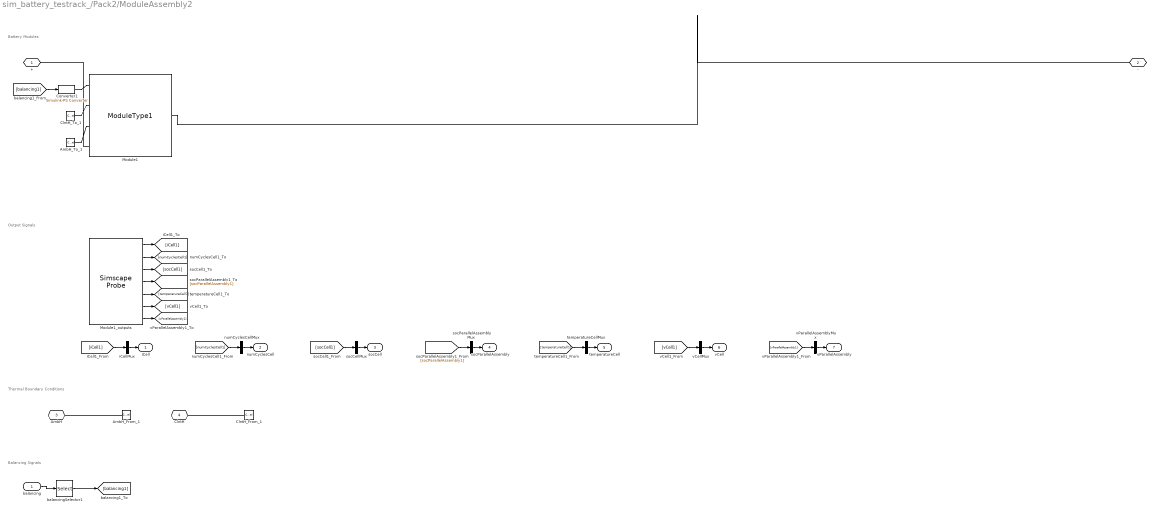
== system sim_battery_testrack_/Pack2/ModuleAssembly2 ==
  note: Balancing Signals
  note: Thermal Boundary Conditions
  note: Output Signals
  note: Battery Modules
  balancing : Inport  PortDimensions=14
  AmbH_From_1 : ConnectionLabel  Label=ambH_1
  AmbH_To_1 : ConnectionLabel  Label=ambH_1
  ClntH_From_1 : ConnectionLabel  Label=clntH_1
  ClntH_To_1 : ConnectionLabel  Label=clntH_1
  Converter1 : nesl_utility/Simulink-PS Converter  PhysicalDomain=network_engine_domain  SubClassName=ps_input  LeftPortType=input  RightPortType=output  PseudoPeriodic=off  Frequencies=[]  NoiseDistribution=none  NoiseParameters=[]  Unit=1  AffineConversion=off  FilteringAndDerivatives=provide  SimscapeFilterOrder=1  InputFilterTimeConstant=0.001  UdotUserProvided=0
  Module1 : GD_Batterymodel_6_lib/Modules/ModuleType1  SOC_vecCell=ModuleType1.SOC_vecCell  T_vecCell=ModuleType1.T_vecCell K  V0_matCell=ModuleType1.V0_matCell V  V_rangeCell=ModuleType1.V_rangeCell V  R0_matCell=ModuleType1.R0_matCell Ohm  AHCell=ModuleType1.AHCell A*hr  extrapolation_optionCell=simscape.enum.extrapolation.nearest  R1_matCell=ModuleType1.R1_matCell Ohm  tau1_matCell=ModuleType1.tau1_matCell s  R2_matCell=ModuleType1.R2_matCell Ohm  tau2_matCell=ModuleType1.tau2_matCell s  thermal_massCell=ModuleType1.thermal_massCell J/K  CoolantResistance=ModuleType1.CoolantResistance K/W  AmbientResistance=ModuleType1.AmbientResistance K/W  CellBalancingClosedResistance=ModuleType1.CellBalancingClosedResistance Ohm  CellBalancingOpenConductance=ModuleType1.CellBalancingOpenConductance 1/Ohm  CellBalancingThreshold=ModuleType1.CellBalancingThreshold  CellBalancingResistance=ModuleType1.CellBalancingResistance Ohm  P=3  S=14  iCell_specify=on  iCell_priority=None  iCell=ModuleAssembly2.Module1.iCell A  iCell_nominal_specify=off  iCell_nominal_unit=A  iCell_nominal_value=1  vCell_specify=on  vCell_priority=None  vCell=ModuleAssembly2.Module1.vCell V  vCell_nominal_specify=off  vCell_nominal_unit=V  vCell_nominal_value=1  socCell_specify=on  socCell_priority=High  socCell=ModuleAssembly2.Module1.socCell  socCell_nominal_specify=off  socCell_nominal_unit=1  socCell_nominal_value=1  numCyclesCell_specify=on  numCyclesCell_priority=High  numCyclesCell=ModuleAssembly2.Module1.numCyclesCell  numCyclesCell_nominal_specify=off  numCyclesCell_nominal_unit=1  numCyclesCell_nominal_value=1  temperatureCell_specify=on  temperatureCell_priority=High  temperatureCell=ModuleAssembly2.Module1.temperatureCell K  temperatureCell_nominal_specify=off  temperatureCell_nominal_unit=K  temperatureCell_nominal_value=1  vParallelAssembly_specify=on  vParallelAssembly_priority=None  vParallelAssembly=ModuleAssembly2.Module1.vParallelAssembly V  vParallelAssembly_nominal_specify=off  vParallelAssembly_nominal_unit=V  vParallelAssembly_nominal_value=1  socParallelAssembly_specify=on  socParallelAssembly_priority=None  socParallelAssembly=ModuleAssembly2.Module1.socParallelAssembly  socParallelAssembly_nominal_specify=off  socParallelAssembly_nominal_unit=1  socParallelAssembly_nominal_value=1
      settings: InternalSimscapePortConfiguration="{\"Bottom\":[{\"id\":\"n\",\"label\":\"-\",\"type\":\"foundation.electrical.electrical\"}],\"Left\":[{\"id\":\"enableCellBalancing\",\"label\":\"CB\",\"type\":\"input\"},{\"id\":\"ClntH\",\"label\":\"CH\",\"type\":\"foundation.thermal.thermal\"},{\"id\":\"AmbH\",\"label\":\"AH\",\"type\":\"foundation.thermal.thermal\"}],\"Right\":[],\"Top\":[{\"id\":\"p\",\"label\":\"+\",\"type\":\"foundation.electrical.electrical\"}]}"
  Module1_outputs : SimscapeProbe  BoundBlock=1428  Variables={iCell, numCyclesCell, socCell, socParallelAssembly, temperatureCell, vCell, vParallelAssembly}
  balancingSelector1 : Selector  InputPortWidth=14  IndexOptions=Index vector (dialog)  Indices="[1   2   3   4   5   6   7   8   9  10  11  12  13  14]"  OutputSizes=1
  iCellMux : Mux  Inputs=1
  numCyclesCellMux : Mux  Inputs=1
  socCellMux : Mux  Inputs=1
  socParallelAssemblyMux : Mux  Inputs=1
  temperatureCellMux : Mux  Inputs=1
  vCellMux : Mux  Inputs=1
  vParallelAssemblyMux : Mux  Inputs=1
  + : PMIOPort  Side=Left
  - : PMIOPort  Port=2  Side=Right
  AmbH : PMIOPort  Port=3  Side=Right  ConnectionType=Connection: foundation.thermal.thermal
  ClntH : PMIOPort  Port=4  Side=Right  ConnectionType=Connection: foundation.thermal.thermal
  iCell : Outport
  numCyclesCell : Outport  Port=2
  socCell : Outport  Port=3
  socParallelAssembly : Outport  Port=4
  temperatureCell : Outport  Port=5
  vCell : Outport  Port=6
  vParallelAssembly : Outport  Port=7
  wires:
  balancingSelector1/1 -> [balancing1]
  balancing/1 -> balancingSelector1/1
  [balancing1] -> Converter1/1
  [vParallelAssembly1] -> vParallelAssemblyMux/1
  vParallelAssemblyMux/1 -> vParallelAssembly/1
  Module1_outputs/7 -> [vParallelAssembly1]
  [vCell1] -> vCellMux/1
  vCellMux/1 -> vCell/1
  Module1_outputs/6 -> [vCell1]
  [temperatureCell1] -> temperatureCellMux/1
  temperatureCellMux/1 -> temperatureCell/1
  Module1_outputs/5 -> [temperatureCell1]
  [socParallelAssembly1] -> socParallelAssemblyMux/1
  socParallelAssemblyMux/1 -> socParallelAssembly/1
  Module1_outputs/4 -> [socParallelAssembly1]
  [socCell1] -> socCellMux/1
  socCellMux/1 -> socCell/1
  Module1_outputs/3 -> [socCell1]
  [numCyclesCell1] -> numCyclesCellMux/1
  numCyclesCellMux/1 -> numCyclesCell/1
  Module1_outputs/2 -> [numCyclesCell1]
  [iCell1] -> iCellMux/1
  iCellMux/1 -> iCell/1
  Module1_outputs/1 -> [iCell1]
  connections:
  Converter1/RConn1 -- Module1/LConn1
  ClntH_From_1/LConn1 -- ClntH/RConn1
  ClntH_To_1/LConn1 -- Module1/LConn2
  AmbH_From_1/LConn1 -- AmbH/RConn1
  AmbH_To_1/LConn1 -- Module1/LConn3
  Module1/RConn1 -- -/RConn1
  Module1/LConn4 -- +/RConn1
